simulink model "CoSimulation"  (R2021b)
settings: Solver=FixedStepDiscrete  StartTime=0.0  StopTime=10.0  FixedStep=0.001  RelTol=1e-3
settings Model: Creator=tin.rabuzin  LastModifiedBy=tin.rabuzin

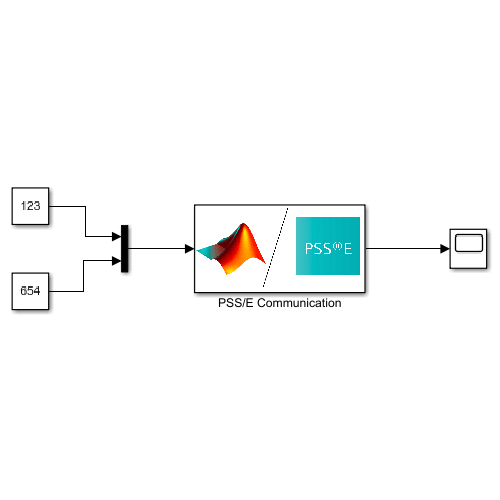
[thumbnail: Simulink's stored preview of the top-level diagram]
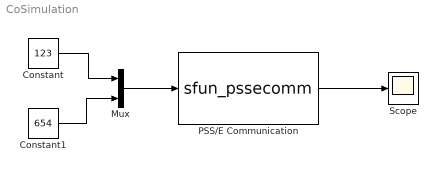
== system CoSimulation ==
  Constant : Constant  Value=123
  Constant1 : Constant  Value=654
  Mux : Mux  Inputs=2
  PSS/E Communication : S-Function  FunctionName=sfun_pssecomm  Parameters=stepsize  SFunctionDeploymentMode=off  EnableBusSupport=off  mask{stepsize=0.001}
      mask prompts: stepsize "Communication step size:"
      mask DialogControl DescGroupVar Prompt: PSS/E Communication Block
      mask DialogControl DescTextVar Prompt: This block sends its block's inputs to PSS/E while the ouputs are what it receives from PSS/E.
      mask Display: image('PSSEComm.png');
  Scope : Scope
  wires:
  Mux/1 -> PSS/E Communication/1
  Constant/1 -> Mux/1
  Constant1/1 -> Mux/2
  PSS/E Communication/1 -> Scope/1
